simulink model "pid_controller"  (R2017a)
settings: Solver=ode4  StartTime=0.0  StopTime=7  FixedStep=10^-3  RelTol=1e-3
settings Model: Creator=Sean  LastModifiedBy=Sean

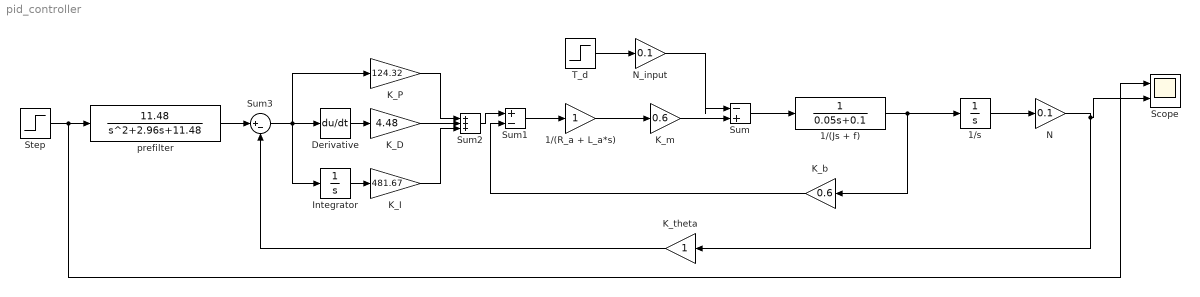
== system pid_controller ==
  1/(Js + f) : TransferFcn  Denominator=[0.05 0.1]
  1/(R_a + L_a*s) : Gain
  1/s : Integrator
  Derivative : Derivative
  Integrator : Integrator
  K_D : Gain  Gain=4.48
  K_I : Gain  Gain=481.67
  K_P : Gain  Gain=124.32
  K_b : Gain  Gain=0.6
  K_m : Gain  Gain=0.6
  K_theta : Gain
  N : Gain  Gain=0.1
  N_input : Gain  Gain=0.1
  Scope : Scope  NumInputPorts=2
  Step : Step  SampleTime=0
  Sum : Sum  Inputs=|-+
  Sum1 : Sum  Inputs=|+-
  Sum2 : Sum  Inputs=+++
  Sum3 : Sum  Inputs=|+-
  T_d : Step  Time=3  After=120  SampleTime=0
  prefilter : TransferFcn  Numerator=[11.48]  Denominator=[1 2.96 11.48]
  wires:
  N/1 -> Scope/2, K_theta/1
  K_theta/1 -> Sum3/2
  K_D/1 -> Sum2/2
  Sum/1 -> 1/(Js + f)/1
  Sum3/1 -> Integrator/1, K_P/1, Derivative/1
  Derivative/1 -> K_D/1
  Sum2/1 -> Sum1/1
  K_b/1 -> Sum1/2
  T_d/1 -> N_input/1
  Sum1/1 -> 1/(R_a + L_a*s)/1
  1/s/1 -> N/1
  K_P/1 -> Sum2/1
  1/(R_a + L_a*s)/1 -> K_m/1
  K_m/1 -> Sum/2
  1/(Js + f)/1 -> K_b/1, 1/s/1
  Integrator/1 -> K_I/1
  K_I/1 -> Sum2/3
  N_input/1 -> Sum/1
  Step/1 -> Scope/1, prefilter/1
  prefilter/1 -> Sum3/1
